simulink model "hengcezhoufangzhen"  (R2012b)
settings: Solver=ode3  StartTime=0.0  StopTime=20  FixedStep=0.005  RelTol=1e-3
settings Model: Creator=Administrator  LastModifiedBy=Administrator

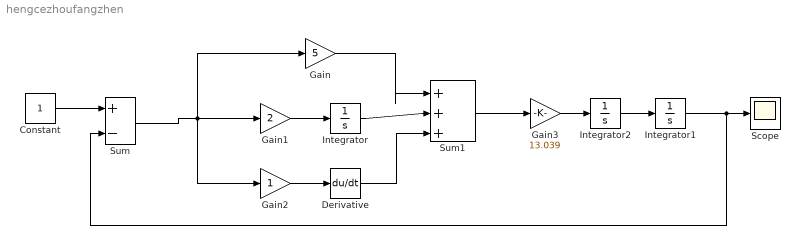
== system hengcezhoufangzhen ==
  Constant : Constant
  Derivative : Derivative
  Gain : Gain  Gain=5
  Gain1 : Gain  Gain=2
  Gain2 : Gain
  Gain3 : Gain  Gain=13.039
  Integrator : Integrator
  Integrator1 : Integrator
  Integrator2 : Integrator
  Scope : Scope
      settings: MaxDataPoints=5000000
  Sum : Sum  Inputs=+-
  Sum1 : Sum  Inputs=|+++
  wires:
  Constant/1 -> Sum/1
  Sum/1 -> Gain/1, Gain2/1, Gain1/1
  Gain1/1 -> Integrator/1
  Gain2/1 -> Derivative/1
  Gain/1 -> Sum1/1
  Integrator/1 -> Sum1/2
  Derivative/1 -> Sum1/3
  Sum1/1 -> Gain3/1
  Gain3/1 -> Integrator2/1
  Integrator2/1 -> Integrator1/1
  Integrator1/1 -> Scope/1, Sum/2
